simulink model "asbCubeSatACS"  (R2025b)
settings: Solver=FixedStepDiscrete  StartTime=0.0  StopTime=10.0  FixedStep=CubeSatTimeStep  RelTol=1e-3  EnableMultiTasking=on
undefined symbols (not defined in the file): gains
libraries: aerolibsatdyn x2, aerolibutil x2, sharedtransform x2, slpidlib x1
settings Model: DataDictionary=asbCubeSatModelData.sldd  ExtModeAutoUpdateStatusClock=off  Creator=The MathWorks, Inc.  LastModifiedBy=excal
settings SolverCC: AlgebraicLoopSolver=TrustRegion  MaxZcPerStep=1.0
settings DataIOCC: LimitDataPoints=on  SaveFormat=Array  SaveOutput=off  SignalLogging=off  DSMLogging=off  SaveTime=off  ReturnWorkspaceOutputs=off
settings OptimizationCC: DefaultParameterBehavior=Inlined  OptimizeBlockIOStorage=off  BufferReuse=off  GlobalBufferReuse=off  ExpressionFolding=off  ExpressionDepthLimit=2147483647.0  LocalBlockOutputs=off  InitFltsAndDblsToZero=on  LifeSpan=inf  OptimizeDataStoreBuffers=off  BusAssignmentInplaceUpdate=off
settings DebuggingCC: ArtificialAlgebraicLoopMsg=none  SolverPrmCheckMsg=warning  FcnCallInpInsideContextMsg=warning  UnconnectedInputMsg=warning  UnconnectedOutputMsg=warning  UnconnectedLineMsg=warning  StateNameClashWarn=warning  PregeneratedLibrarySubsystemCodeDiagnostic=none  SFUnexpectedBacktrackingDiag=warning  SFNoUnconditionalDefaultTransitionDiag=warning  SFExecutionAtInitializationDiag=none  ArithmeticOperatorsInVariantConditions=warning
settings HardwareCC: ProdBitPerPointer=32.0  ProdBitPerSizeT=32.0  ProdBitPerPtrDiffT=32.0  ProdLargestAtomicFloat=None  ProdIntDivRoundTo=Undefined  ProdEndianess=Unspecified  ProdWordSize=32.0  ProdHWDeviceType=32-bit Generic
settings ModelReferenceCC: EnableRefExpFcnMdlSchedulingChecks=on  PropagateSignalLabelsOutOfModel=off
settings SFSimCC: SimUseLocalCustomCode=off
settings RTWCC: RTWUseLocalCustomCode=off  GPUComputeCapability=3.5  DLArmComputeVersion=19.05
settings CodeAppCC: StateflowObjectComments=on
settings GRTTargetCC: TargetFcnLib=ansi_tfl_tmw.mat  TargetLangStandard=C89/C90 (ANSI)  CombineOutputUpdateFcns=off  GRTInterface=on
settings ConfigComp: CovMetricSettings=dw  CovSaveCumulativeToWorkspaceVar=on  CovSaveSingleToWorkspaceVar=on  CovExternalEMLEnable=off

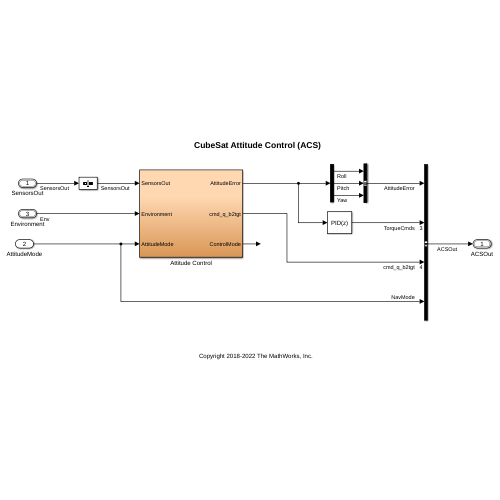
[thumbnail: Simulink's stored preview of the top-level diagram]
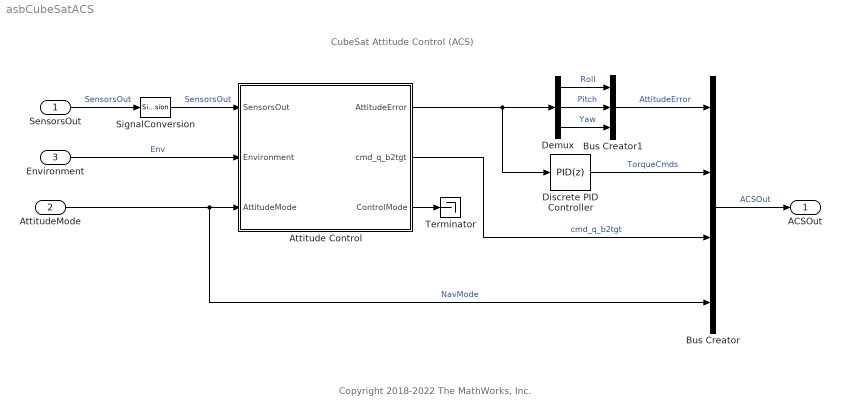
== system asbCubeSatACS ==
  note: Copyright 2018-2022 The MathWorks, Inc.
  note: CubeSat Attitude Control (ACS)
  SensorsOut : Inport  OutDataTypeStr=Bus: StatesOutBus
  AttitudeMode : Inport  Port=2  OutDataTypeStr=double  PortDimensions=1
  Environment : Inport  Port=3  OutDataTypeStr=Bus: EnvBus  PortDimensions=1
  Attitude Control : Subsystem
  Bus Creator : BusCreator  Inputs=4  OutDataTypeStr=Bus: ACSOutBus  NonVirtualBus=on
  Bus Creator1 : BusCreator  Inputs=3  OutDataTypeStr=Bus: AttitudeErrorBus
  Demux : Demux  Outputs=3
  Discrete PID Controller : slpidlib/PID Controller  Controller=PID  Form=Parallel  TimeDomain=Discrete-time  UseExternalTs=off  SampleTime=-1  IntegratorMethod=Forward Euler  FilterMethod=Forward Euler  ControllerParametersSource=internal  P=gains.Kp  I=gains.Ki  UseKiTs=off  D=gains.Kd  UseExternalDerivativeSource=off  N=1000  UseFilter=off  TunerSelectOption=Transfer Function Based (PID Tuner App)  InitialConditionSource=internal  InitialConditionForIntegrator=0  InitialConditionForFilter=0  DifferentiatorICPrevScaledInput=0  ExternalReset=none  TrackingMode=off  Kt=1  LimitOutput=off  SatLimitsSource=internal  UpperSaturationLimit=inf  LowerSaturationLimit=-inf  LinearizeAsGain=off  AntiWindupMode=none  Kb=1  LimitIntegrator=off  UpperIntegratorSaturationLimit=inf  LowerIntegratorSaturationLimit=-inf  POutMin=[]  POutMax=[]  IOutMin=[]  IOutMax=[]  DOutMin=[]  DOutMax=[]  NOutMin=[]  NOutMax=[]  SumOutMin=[]  SumOutMax=[]  SaturationOutMin=[]  SaturationOutMax=[]  PParamMin=[]  PParamMax=[]  IParamMin=[]  IParamMax=[]  DParamMin=[]  DParamMax=[]  NParamMin=[]  NParamMax=[]  KbParamMin=[]  KbParamMax=[]  KtParamMin=[]  KtParamMax=[]  KbOutMin=[]  KbOutMax=[]  KtOutMin=[]  KtOutMax=[]  IntegratorOutMin=[]  IntegratorOutMax=[]  FilterOutMin=[]  FilterOutMax=[]  SumI1OutMin=[]  SumI1OutMax=[]  SumI2OutMin=[]  SumI2OutMax=[]  SumI3OutMin=[]  SumI3OutMax=[]  SumI4OutMin=[]  SumI4OutMax=[]  SumDOutMin=[]  SumDOutMax=[]  DifferentiatorOutMin=[]  DifferentiatorOutMax=[]  FilterDiffOutCoefMin=[]  FilterDiffOutCoefMax=[]  ReciprocalOutMin=[]  ReciprocalOutMax=[]  SumDenOutMin=[]  SumDenOutMax=[]  SumNumOutMin=[]  SumNumOutMax=[]  DivideOutMin=[]  DivideOutMax=[]  UdiffTsProdOutMin=[]  UdiffTsProdOutMax=[]  NTsProdOutMin=[]  NTsProdOutMax=[]  UintegralTsProdOutMin=[]  UintegralTsProdOutMax=[]  UngainTsProdOutMin=[]  UngainTsProdOutMax=[]  ClampingZeroOutDataTypeStr=Inherit: Inherit via back propagation  ClampingZeroOutMin=[]  ClampingZeroOutMax=[]  FilterDenConstantOutDataTypeStr=Inherit: Inherit via back propagation  FilterDenConstantOutMin=[]  FilterDenConstantOutMax=[]  PCopyOutDataTypeStr=Inherit: Inherit via back propagation  PCopyOutMin=[]  PCopyOutMax=[]  NCopyOutDataTypeStr=Inherit: Inherit via back propagation  NCopyOutMin=[]  NCopyOutMax=[]  IntegratorContinuousStateAttributes=''  IntegratorStateMustResolveToSignalObject=off  IntegratorRTWStateStorageClass=Auto  FilterContinuousStateAttributes=''  FilterStateMustResolveToSignalObject=off  FilterRTWStateStorageClass=Auto  ParallelPVariant=InternalParameters  IdealPVariant=Disabled  IVariant=InternalParameters  DVariant=InternalParameters  IntegratorVariant=Discrete  SatVariant=Disabled  AWVariant=Passthrough  PCopyVariant=Disabled  TRVariant=Disabled  FdbkBlocksVariant=Forward  IdealPFdbkVariant=Disabled  SatFdbkVariant=Disabled  DerivativeFilterVariant=Differentiator  NVariant=Passthrough  NCopyVariant=Disabled_SignalSpec  FilterICVariant=InternalICsDifferentiator  IntegratorICVariant=InternalICs  ExternalResetVariant=Disabled  TRSumVariant=Passthrough  SumFdbkVariant=Disabled  SumVariant=Sum_PID  TsampFilterVariant=InternalTs  TsampNgainVariant=Passthrough  TsampIntegralVariant=Disabled_SignalSpec  ExternalSaturationOutDataTypeStr=Inherit: Same as second input  DerivativeSourceVariant=ErrorSignal  PreIntVariant=InternalPreInt
  SignalConversion : SignalConversion  ConversionOutput=Virtual bus  OverrideOpt=off
  Terminator : Terminator
  ACSOut : Outport  OutDataTypeStr=Bus: ACSOutBus  PortDimensions=1  VectorParamsAs1DForOutWhenUnconnected=off  BusOutputAsStruct=on
  wires:
  Demux/1 -> Bus Creator1/1  "Roll"
  AttitudeMode/1 -> Bus Creator/4, Attitude Control/3("AttitudeMode ")  "NavMode"
  Demux/2 -> Bus Creator1/2  "Pitch"
  SensorsOut/1 -> SignalConversion/1  "SensorsOut"
  Bus Creator1/1 -> Bus Creator/1  "AttitudeError"
  Demux/3 -> Bus Creator1/3  "Yaw"
  Discrete PID Controller/1 -> Bus Creator/2  "TorqueCmds"
  Bus Creator/1 -> ACSOut/1  "ACSOut"
  Attitude Control/1(AttitudeError) -> Discrete PID Controller/1, Demux/1
  Attitude Control/3(" ControlMode") -> Terminator/1
  Environment/1 -> Attitude Control/2(Environment)  "Env"
  Attitude Control/2(cmd_q_b2tgt) -> Bus Creator/3  "cmd_q_b2tgt"
  SignalConversion/1 -> Attitude Control/1("SensorsOut ")  "SensorsOut"

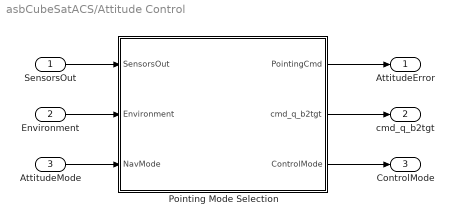
== system asbCubeSatACS/Attitude Control ==
  "SensorsOut " : Inport  OutDataTypeStr=Bus: StatesOutBus
  Environment : Inport  Port=2
  "AttitudeMode " : Inport  Port=3
  Pointing Mode Selection : Stateflow chart  RequirementInfo="{}  %GIDa_a065c7c8_537d_4123_b3cc_6e7e7008a32c"  TreatAsAtomicUnit=on
  AttitudeError : Outport  VectorParamsAs1DForOutWhenUnconnected=off
  cmd_q_b2tgt : Outport  Port=2  VectorParamsAs1DForOutWhenUnconnected=off
  " ControlMode" : Outport  Port=3  VectorParamsAs1DForOutWhenUnconnected=off
  wires:
  "SensorsOut "/1 -> Pointing Mode Selection/1(SensorsOut)
  Pointing Mode Selection/3(ControlMode) -> " ControlMode"/1
  "AttitudeMode "/1 -> Pointing Mode Selection/3(NavMode)
  Environment/1 -> Pointing Mode Selection/2(Environment)
  Pointing Mode Selection/1(PointingCmd) -> AttitudeError/1
  Pointing Mode Selection/2(cmd_q_b2tgt) -> cmd_q_b2tgt/1

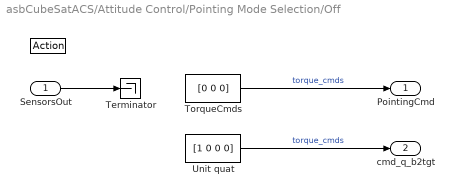
== system asbCubeSatACS/Attitude Control/Pointing Mode Selection/Off ==
  SensorsOut : Inport  OutDataTypeStr=Bus: StatesOutBus
  " " : ActionPort
      settings: CopyFcn=Stateflow.SLINSF.SimulinkMan.removeBlockPreDeleteFcn  PreDeleteFcn=Stateflow.SLINSF.SimulinkMan.unsafePredeleteFcn
  Terminator : Terminator
  TorqueCmds : Constant  Value=[0 0 0]
  Unit quat : Constant  Value=[1 0 0 0]
  PointingCmd : Outport  RequirementInfo="{}  %GIDa_4dc055f9_6cac_42e1_8ddb_4145586b89f5"  VectorParamsAs1DForOutWhenUnconnected=off
  cmd_q_b2tgt : Outport  RequirementInfo="{}  %GIDa_ca05d0a6_a581_4c3e_b3a0_cd281b586de8"  Port=2  VectorParamsAs1DForOutWhenUnconnected=off
  wires:
  SensorsOut/1 -> Terminator/1
  TorqueCmds/1 -> PointingCmd/1  "torque_cmds"
  Unit quat/1 -> cmd_q_b2tgt/1  "torque_cmds"

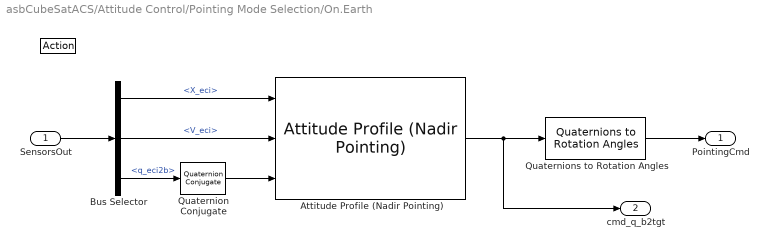
== system asbCubeSatACS/Attitude Control/Pointing Mode Selection/On.Earth ==
  SensorsOut : Inport  OutDataTypeStr=Bus: StatesOutBus
  " " : ActionPort
      settings: CopyFcn=Stateflow.SLINSF.SimulinkMan.removeBlockPreDeleteFcn  PreDeleteFcn=Stateflow.SLINSF.SimulinkMan.unsafePredeleteFcn
  Attitude Profile (Nadir Pointing) : aerolibsatdyn/Attitude Profile (Nadir Pointing)  outputError=on  outputFinalAttitude=off  portFrame=ICRF  pointingMode=Point at nadir  celestialTarget=Sun  tunablePointing=off  primaryAlignmentSrc=Dialog  primaryAlignment=[0 0 1]  secondaryAlignmentSrc=Dialog  secondaryAlignment=[1 0 0]  constraintFrame=LVLH  primaryConstraintSrc=Dialog  primaryConstraint=[1 0 0]  secondaryConstraintSrc=Dialog  secondaryConstraint=[0 1 0]
  Bus Selector : BusSelector  OutputSignals=X_eci,V_eci,q_eci2b
  Quaternion Conjugate : aerolibutil/Quaternion Conjugate
  Quaternions to Rotation Angles : sharedtransform/Quaternions to Rotation Angles  rotationOrder=XYZ  aMode=aMode
  PointingCmd : Outport  VectorParamsAs1DForOutWhenUnconnected=off
  cmd_q_b2tgt : Outport  RequirementInfo="{}  %GIDa_69a01501_0b6a_41cf_b570_f5b49bb229cd"  Port=2  VectorParamsAs1DForOutWhenUnconnected=off
  wires:
  Quaternions to Rotation Angles/1 -> PointingCmd/1
  Bus Selector/3 -> Quaternion Conjugate/1  "<q_eci2b>"
  Bus Selector/2 -> Attitude Profile (Nadir Pointing)/2  "<V_eci>"
  SensorsOut/1 -> Bus Selector/1
  Bus Selector/1 -> Attitude Profile (Nadir Pointing)/1  "<X_eci>"
  Quaternion Conjugate/1 -> Attitude Profile (Nadir Pointing)/3
  Attitude Profile (Nadir Pointing)/1 -> cmd_q_b2tgt/1, Quaternions to Rotation Angles/1

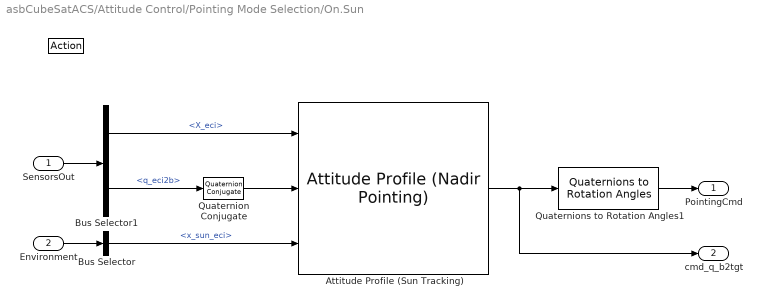
== system asbCubeSatACS/Attitude Control/Pointing Mode Selection/On.Sun ==
  SensorsOut : Inport  OutDataTypeStr=Bus: StatesOutBus
  Environment : Inport  Port=2  OutDataTypeStr=Bus: EnvBus
  " " : ActionPort
      settings: CopyFcn=Stateflow.SLINSF.SimulinkMan.removeBlockPreDeleteFcn  PreDeleteFcn=Stateflow.SLINSF.SimulinkMan.unsafePredeleteFcn
  Attitude Profile (Sun Tracking) : aerolibsatdyn/Attitude Profile (Nadir Pointing)  outputError=on  outputFinalAttitude=off  portFrame=ICRF  pointingMode=Custom  celestialTarget=Sun  tunablePointing=off  primaryAlignmentSrc=Dialog  primaryAlignment=[0 0 -1]  secondaryAlignmentSrc=Dialog  secondaryAlignment=[1 0 0]  constraintFrame=ICRF  primaryConstraintSrc=Port  primaryConstraint=[1 0 0]  secondaryConstraintSrc=Dialog  secondaryConstraint=[0 0 1]
  Bus Selector : BusSelector  OutputSignals=x_sun_eci
  Bus Selector1 : BusSelector  OutputSignals=X_eci,q_eci2b
  Quaternion Conjugate : aerolibutil/Quaternion Conjugate
  Quaternions to Rotation Angles1 : sharedtransform/Quaternions to Rotation Angles  rotationOrder=XYZ  aMode=aMode
  PointingCmd : Outport  VectorParamsAs1DForOutWhenUnconnected=off
  cmd_q_b2tgt : Outport  Port=2  VectorParamsAs1DForOutWhenUnconnected=off
  wires:
  Attitude Profile (Sun Tracking)/1 -> Quaternions to Rotation Angles1/1, cmd_q_b2tgt/1
  SensorsOut/1 -> Bus Selector1/1
  Environment/1 -> Bus Selector/1
  Quaternions to Rotation Angles1/1 -> PointingCmd/1
  Bus Selector/1 -> Attitude Profile (Sun Tracking)/3  "<x_sun_eci>"
  Quaternion Conjugate/1 -> Attitude Profile (Sun Tracking)/2
  Bus Selector1/2 -> Quaternion Conjugate/1  "<q_eci2b>"
  Bus Selector1/1 -> Attitude Profile (Sun Tracking)/1  "<X_eci>"

== stateflow chart asbCubeSatACS/Attitude Control/Pointing Mode Selection ==
  state On
    state Transition
    state Earth
    state Sun
    (default) -> Transition
    Transition -> Earth [order 1] : [NavMode == 1]
        | {ControlMode = 2;}
    Earth -> Transition : [NavMode == 2]
        | {ControlMode = 1;}
    Transition -> Sun [order 2] : [NavMode == 2]
        | {ControlMode = 2;}
    Sun -> Transition : [NavMode == 1]
        | {ControlMode = 1;}
  state Off
  (default) -> Off
  Off -> On : [NavMode ~= 0]
      | {ControlMode = 1;}
  On -> Off : [NavMode == 0]
      | {ControlMode = 0;}
  data: sf_internal_action_state_placeholder_data local double size=1 =0; sf_internal_action_state_placeholder_data local double size=1 =0; sf_internal_action_state_placeholder_data local double size=1 =0; SensorsOut input Bus: StatesOutBus; Environment input; NavMode input; PointingCmd output =[0 0 0]'; cmd_q_b2tgt output; ControlMode output
